simulink model "analisando_espectro"  (R2015a)
settings: Solver=ode45  StartTime=0.0  StopTime=10.0  RelTol=1e-3
undefined symbols (not defined in the file): a1, f1, fa, Ta
libraries: dspsrcs4 x3, dsparch4 x1, dspsnks4 x1
settings Model: Creator=aluno  LastModifiedBy=aluno

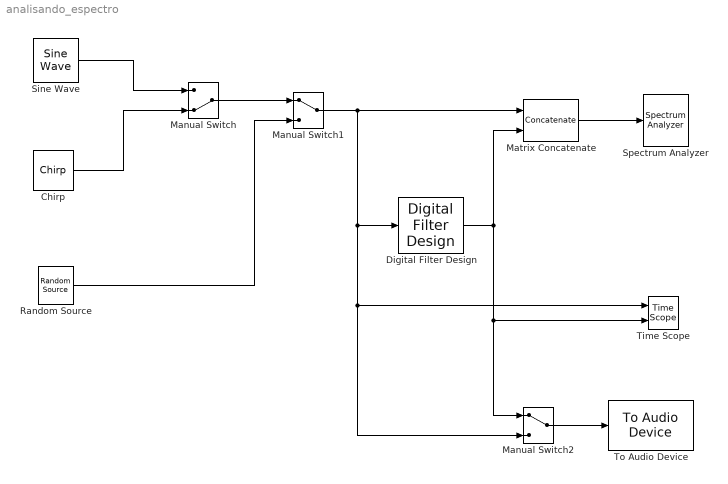
== system analisando_espectro ==
  Chirp : dspsrcs4/Chirp  sweep=Linear  mode=Unidirectional  f0=0  f1=fa/2  t1=4  Tsweep=4  phase=0  Ts=Ta  spf=spf  datatype=Double
  Digital Filter Design : dsparch4/Digital Filter Design  mwdsp_browser_bugfix_var=off
  Manual Switch : ManualSwitch  CurrentSetting=0
  Manual Switch1 : ManualSwitch
  Manual Switch2 : ManualSwitch
  Matrix Concatenate : Concatenate  Mode=Multidimensional array  ConcatenateDimension=2
  Random Source : dspsrcs4/Random Source  SrcType=Uniform  NormMethod=Ziggurat  CltLength=12  MinVal=-1  MaxVal=1  MeanVal=0  VarVal=1  RepMode=Not repeatable  rawSeed=1  IsInherit=off  SampMode=Discrete  SampTime=Ta  SampFrame=spf  DataType=Double  OutComplex=Real
  Sine Wave : dspsrcs4/Sine Wave  Amplitude=a1  Frequency=f1  Phase=0  SampleMode=Discrete  OutComplex=Real  CompMethod=Trigonometric fcn  TableSize=Speed  SampleTime=Ta  SamplesPerFrame=spf  ResetState=Restart at time zero  dataType=double  wordLen=16  udDataType=sfix(16)  fracBitsMode=Best precision  numFracBits=15  OutDataTypeStr=double  LastOutDataTypeStr=double
  Spectrum Analyzer : SpectrumAnalyzer
  Time Scope : TimeScope  DefaultConfigurationName=spbscopes.TimeScopeBlockCfg  NumInputPorts=2
  To Audio Device : dspsnks4/To Audio Device  deviceName=Default  inheritSampleRate=on  sampleRate=44100  deviceDatatype=Determine from input data type  autoBufferSize=on  bufferSize=4096  queueDuration=1.0  defaultOutputChannelMapping=on  outputChannelMapping=1:2  outputNumUnderrunSamples=off
  wires:
  Sine Wave/1 -> Manual Switch/1
  Chirp/1 -> Manual Switch/2
  Manual Switch/1 -> Manual Switch1/1
  Random Source/1 -> Manual Switch1/2
  Manual Switch1/1 -> Digital Filter Design/1, Time Scope/1, Manual Switch2/2, Matrix Concatenate/1
  Matrix Concatenate/1 -> Spectrum Analyzer/1
  Manual Switch2/1 -> To Audio Device/1
  Digital Filter Design/1 -> Manual Switch2/1, Time Scope/2, Matrix Concatenate/2
